simulink model "pipline_system"  (R2022b)
settings: Solver=FixedStepAuto  StartTime=0.0  StopTime=t_sim_stop  FixedStep=Ts  RelTol=1e-5
values from neighbouring files (symbols this model uses):
  A_inv = pinv(Ad-eye(n),0.01)    [run_pipeline_system.m]
  Aeq = [A_bar -B_bar ... (first row only)    [run_pipeline_system.m]
  B = -[1;0;0;0]    [run_pipeline_system.m]
  B_dem = -[0;0;0;1]    [run_pipeline_system.m]
  B_demd = B_dem*Ts    [run_pipeline_system.m]
  B_h = -[0 0;1 0;0 1;0 0]    [run_pipeline_system.m]
  B_hd = B_h*Ts    [run_pipeline_system.m]
  c = 330    [run_pipeline_system.m]
  h = 10    [run_pipeline_system.m]
  K_inv = (pi^2)/(64*c^2)*f*D_edge.^5./L_edge    [run_pipeline_system.m]
  M = blkdiag(Q_bar, R_bar)    [run_pipeline_system.m]
  n = 4    [run_pipeline_system.m]
  p_eq = [P1;P2;P3;P4]    [run_pipeline_system.m]
  Q = 1e-5    (= 1e-05)    [run_pipeline_system.m]
  R = 1e-5    (= 1e-05)    [run_pipeline_system.m]
  Ts = 0.05    [run_pipeline_system.m]
  V = (pi/8)*sum(((D_edge.^2).*L_edge),2,'omitnan')    [run_pipeline_system.m]
  w_eq = c^2*(sqrt(K_inv.*abs(l*(p_eq.^2).' - (p_eq.^2)*l.')).*sign(l*p_eq.' - p_eq*l.')*l)./V    [run_pipeline_system.m]
libraries: simulink x2, sharedTrackingLibrary x1
settings Model: Creator=Anubi  LastModifiedBy=Abelb
settings HardwareCC: TargetBitPerPointer=64  TargetBitPerSizeT=64  TargetBitPerPtrDiffT=64  TargetLongLongMode=on  TargetIntDivRoundTo=Zero  TargetEndianess=LittleEndian  TargetWordSize=64  TargetHWDeviceType=MATLAB Host  ProdEqTarget=off
settings ModelReferenceCC: EnableRefExpFcnMdlSchedulingChecks=on
settings RTWCC: Description=Rapid Simulation Target  SystemTargetFile=rsim.tlc  TemplateMakefile=rsim_default_tmf
settings RSimTargetCC: TargetLangStandard=C99 (ISO)  OptimizeReductions=off

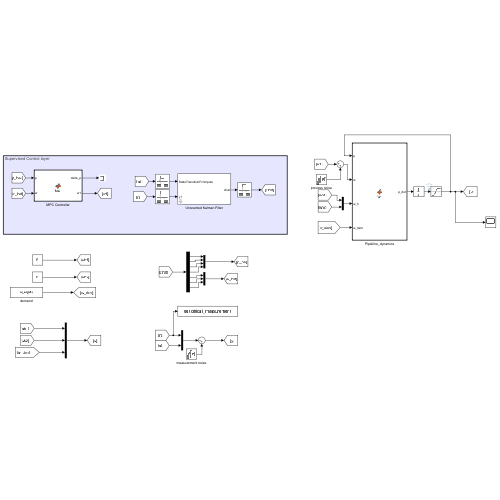
[thumbnail: Simulink's stored preview of the top-level diagram]
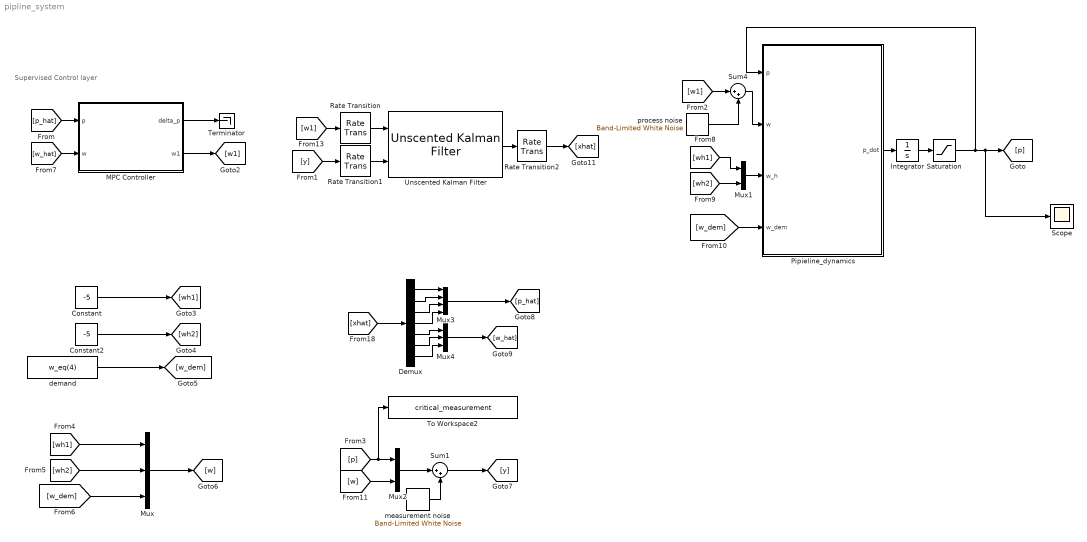
== system pipline_system ==
  note: Supervised Control layer
  Constant : Constant  Value=-5
  Constant2 : Constant  Value=-5
  Demux : Demux  Outputs=7
  Integrator : Integrator  InitialCondition=p_eq
  MPC Controller : MATLAB Function  TreatAsAtomicUnit=on
  Mux : Mux  Inputs=3
  Mux1 : Mux  Inputs=2
  Mux2 : Mux  Inputs=2
  Mux3 : Mux
  Mux4 : Mux  Inputs=3
  Pipieline_dynamics : MATLAB Function  TreatAsAtomicUnit=on
  Rate Transition : RateTransition  InitialCondition=w_eq(1)  OutPortSampleTime=Ts
  Rate Transition1 : RateTransition  InitialCondition=[w_eq(2:end); p_eq]  OutPortSampleTime=Ts
  Rate Transition2 : RateTransition  InitialCondition=[w_eq(2:end); p_eq]  OutPortSampleTime=0
  Saturation : Saturate  UpperLimit=inf  LowerLimit=0
  Scope : Scope
  Sum1 : Sum  Inputs=|++
  Sum4 : Sum  Inputs=|++
  Terminator : Terminator
  To Workspace2 : ToWorkspace  VariableName=critical_measurement  SaveFormat=Timeseries  SampleTime=-1
  Unscented Kalman Filter : sharedTrackingLibrary/Unscented Kalman Filter  StateTransitionFcn=myStateTransitionFcn  HasAdditiveProcessNoise=Additive  ProcessNoise=Q*eye(7)  HasTimeVaryingProcessNoise=off  HasStateTransitionFcnExtraArgument=1  InitialState=[p_eq; w_eq(2:end)]  InitialStateCovariance=1  Alpha=1e-3  Beta=2  Kappa=0  MeasurementFcn1=myMeasurementFcn  HasMeasurementEnablePort1=off  HasAdditiveMeasurementNoise1=Additive  MeasurementNoise1=R*eye(7)  HasTimeVaryingMeasurementNoise1=off  HasMeasurementFcnExtraArgument1=0  HasMeasurementWrapping1=off  MeasurementFcn2=myMeasurementFcn  HasMeasurementEnablePort2=off  HasAdditiveMeasurementNoise2=Additive  MeasurementNoise2=1  HasTimeVaryingMeasurementNoise2=off  HasMeasurementFcnExtraArgument2=0  HasMeasurementWrapping2=off  MeasurementFcn3=myMeasurementFcn  HasMeasurementEnablePort3=off  HasAdditiveMeasurementNoise3=Additive  MeasurementNoise3=1  HasTimeVaryingMeasurementNoise3=off  HasMeasurementFcnExtraArgument3=0  HasMeasurementWrapping3=off  MeasurementFcn4=myMeasurementFcn  HasMeasurementEnablePort4=off  HasAdditiveMeasurementNoise4=Additive  MeasurementNoise4=1  HasTimeVaryingMeasurementNoise4=off  HasMeasurementFcnExtraArgument4=0  HasMeasurementWrapping4=off  MeasurementFcn5=myMeasurementFcn  HasMeasurementEnablePort5=off  HasAdditiveMeasurementNoise5=Additive  MeasurementNoise5=1  HasTimeVaryingMeasurementNoise5=off  HasMeasurementFcnExtraArgument5=0  HasMeasurementWrapping5=off  EnableMultirate=off  StateTransitionFcnSampleTime=1  MeasurementFcn1SampleTime=1  MeasurementFcn2SampleTime=1  MeasurementFcn3SampleTime=1  MeasurementFcn4SampleTime=1  MeasurementFcn5SampleTime=1  UseCurrentEstimator=on  OutputStateCovariance=off  DataType=double  SampleTime=Ts  NumberOfMeasurements=1
      settings: LibrarySourceBlock=cstblocks/State Estimation/Unscented Kalman Filter
  demand : Constant  Value=w_eq(4)
  measurement noise : simulink/Sources/Band-Limited White Noise  Cov=R*Ts  Ts=0.1  seed=[23341]
  process noise : simulink/Sources/Band-Limited White Noise  Cov=R*Ts  Ts=0.1  seed=[23341]
  wires:
  Pipieline_dynamics/1(p_dot) -> Integrator/1
  Integrator/1 -> Saturation/1
  MPC Controller/2(w1) -> [w1]
  demand/1 -> [w_dem]
  Mux1/1 -> Pipieline_dynamics/3(w_h)
  [wh1] -> Mux1/1
  [wh2] -> Mux1/2
  [w_dem] -> Pipieline_dynamics/4(w_dem)
  [wh2] -> Mux/2
  [w_dem] -> Mux/3
  MPC Controller/1(delta_p) -> Terminator/1
  Constant/1 -> [wh1]
  Constant2/1 -> [wh2]
  [wh1] -> Mux/1
  Mux/1 -> [w]
  Sum1/1 -> [y]
  measurement noise/1 -> Sum1/2
  Mux2/1 -> Sum1/1
  [p] -> To Workspace2/1, Mux2/1
  [w] -> Mux2/2
  [w1] -> Sum4/1
  Sum4/1 -> Pipieline_dynamics/2(w)
  process noise/1 -> Sum4/2
  [y] -> Rate Transition1/1
  [w1] -> Rate Transition/1
  Unscented Kalman Filter/1 -> Rate Transition2/1
  Rate Transition/1 -> Unscented Kalman Filter/1
  Rate Transition1/1 -> Unscented Kalman Filter/2
  Rate Transition2/1 -> [xhat]
  [p_hat] -> MPC Controller/1(p)
  [w_hat] -> MPC Controller/2(w)
  Mux4/1 -> [w_hat]
  Demux/6 -> Mux4/2
  Demux/4 -> Mux3/4
  Demux/3 -> Mux3/3
  Demux/1 -> Mux3/1
  Demux/5 -> Mux4/1
  Demux/7 -> Mux4/3
  Demux/2 -> Mux3/2
  [xhat] -> Demux/1
  Mux3/1 -> [p_hat]
  Saturation/1 -> Scope/1, [p], Pipieline_dynamics/1(p)

== matlab function pipline_system/Pipieline_dynamics ==
  data: p input; p_dot output; w input; w_h input; w_dem input; K_inv parameter; c parameter; V parameter; B_h parameter; B_dem parameter; B parameter
function p_dot = fcn(p,w,w_h,w_dem,K_inv, c, V, B_h, B_dem, B)
% COMMENTS HERE

p_sq = p.^2;
l    = ones(length(p),1);  % vector of ones
Psi = sqrt(K_inv.*abs(l*p_sq.' - p_sq*l.')).*sign(l*p.' - p*l.');

p_dot = c^2*(Psi*l)./V + B_h*w_h + B_dem*w_dem + B*w;

== matlab function pipline_system/MPC Controller ==
  data: delta_p output; p input; w input; w1 output; p_eq parameter; w_eq parameter; M parameter; Aeq parameter; B_hd parameter; B_demd parameter; n parameter; h parameter; A_inv parameter
function [delta_p,w1] = fcn(p,w,p_eq, w_eq, M, Aeq, B_hd, B_demd, n, h,A_inv)

% coder.extrinsic('quad_prog_solver');

%% formulate rest MPC parameters
% feedforward term
delta_w = w-w_eq(2:end);
pw = A_inv*(B_hd*delta_w(1:2) + B_demd*delta_w(3));

% additional internal state
delta_p = p-p_eq + pw;

% equality constraint
% beq1 = [Bh_bar -B_dem_bar]*kron(ones(h,1),delta_w);
beq1 = zeros(n*h,1);
beq2 = delta_p;
beq3 = pw;
beq = [beq1; beq2; beq3];

% objective
F = [-M(1:n*(h+1),1:n*(h+1))*kron(ones(h+1,1),pw); zeros(h,1)];

%% call solver
z = zeros(size(M,1),1);   % z = [delta_p; delta_w]
% z(:) = quad_prog_solver(M,F,Aeq,beq);
N = [M Aeq.';
     Aeq zeros(size(Aeq,1))];

N_inv = pinv(N,0.01);
N_inv1 = N_inv(1:size(M,1),:);

z = N_inv1*[-F; beq];

delta_w1 = z(n*h+1);


%% add feedfowward term
w1 = delta_w1 + w_eq(1);
